simulink model "bidirectional_fixcurrent"  (R2016a)
settings: Solver=ode1  StartTime=0.0  StopTime=4  FixedStep=1e-5  RelTol=1e-3
undefined symbols (not defined in the file): Ion, Lithium
libraries: powerlib x12, simulink x4, powerlib_meascontrol x2, electricdrivelib x1
settings Model: Creator=CpmpuMark  LastModifiedBy=VARUN SINGH
settings DataIOCC: LimitDataPoints=on  SaveFormat=Array
settings DebuggingCC: SolverPrmCheckMsg=warning
settings HardwareCC: ProdBitPerPointer=32  ProdLargestAtomicFloat=None  ProdIntDivRoundTo=Undefined  ProdEndianess=Unspecified  ProdWordSize=32  ProdHWDeviceType=32-bit Generic
settings ModelReferenceCC: PropagateSignalLabelsOutOfModel=off
settings ConfigComp: CovSFcnEnable=off

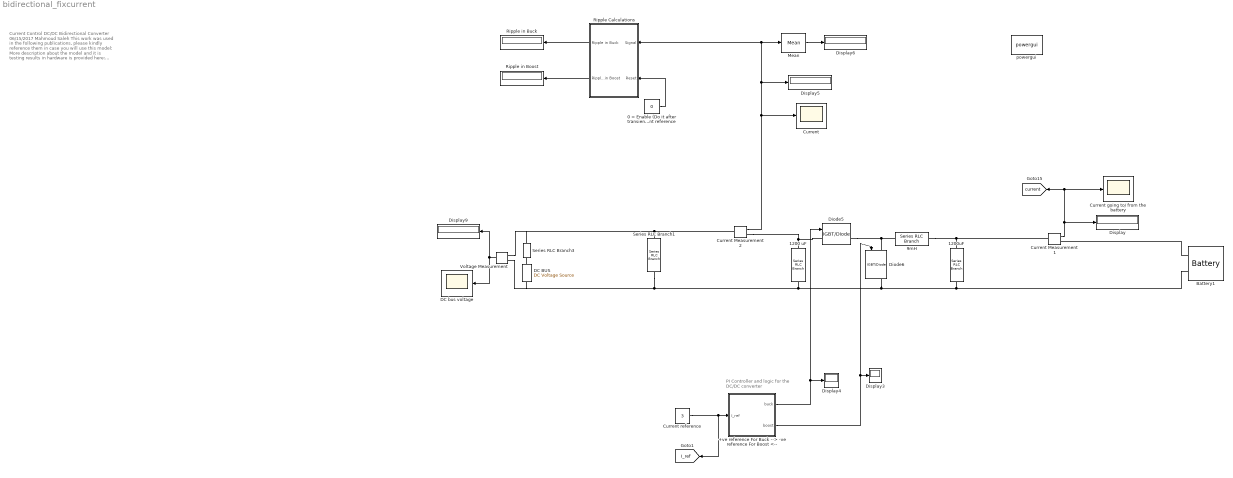
== system bidirectional_fixcurrent ==
  note: Current Control DC/DC Bidirectional Converter
      | 06/15/2017 Mahmoud Saleh
      | This work was used in the following publications, please kindly reference them in case you will use this model:
      |
      | More description about the model and it is testing results in hardware is provided here:
      | http://ieeexplore.ieee.org/document/7454295/
      | OR: https://drive.google.com/open?id=0B7mblFaJhY4VcmZ5OF9ueGxPM1U
      |
      | For Citation use :
      | - M. Saleh , Y. Esa, Y. Mhandi, W. Brandauer and A. Mohamed, "Design and implementation of CCNY DC microgrid testbed,"
      | 2016 IEEE Industry Applications Society Annual Meeting, Portland, OR, 2016.
      |
      | Also This Model was used in the paper:
      | http://ieeexplore.ieee.org/abstract/document/7731870/
      | OR: https://drive.google.com/open?id=0B7mblFaJhY4VY0dXdWdqTWNmUDg
      |
      | For Citation use :
      | -M. Saleh , A. Althaibani, Y. Esa, Y. Mhandi and A. Mohamed, "Impact of clustering microgrids on their stability and resilience during blackouts,"
      | 2015 International Conference on Smart Grid and Clean Energy Technologies (ICSGCE), Offenburg, 2015, pp. 195-200.
      |
      | The description of each element is on top of it and how it was calculated.
      | The model is flexible to work within wide range of values. If you have questions
      | please email me at my main email: mahmoudsah@hotmail.com
      | student email: msaleh000@citymail.cuny,edu
      | gmail: mahmoudsalahem@gmail.com
      | In the subject of your email write: Bidirectional Mathwork question
      | so that I would be able to track the emails even if they went to junk mail.
      | -------------------------------------------
      | I am an expert in modeling in Simulink, especially microgrids, I have encountered
      | many problems and I was able to fix it. I used to work with dSpace and I build with
      | my colleagues microgrid testbed at City College of New York. We modeled according
      | to the hardware components avialable in our lab, then we build it and test it. I
      | will try to help in case you have a question
  note: PI Controller and logic for
      | the DC/DC converter
  +ve reference For Buck --> -ve reference For Boost <-- : Subsystem
  "0 = Enable (Do it after transient, so that it does not calculate ripples during transient) 1 = Reset after every change in current reference" : Constant  Value=0
  1200 uF : powerlib/Elements/Series RLC Branch  LConnTagsString=__new0  RConnTagsString=__new0  BranchType=RC  Resistance=0.1  Inductance=3e-3  SetiL0=off  InitialCurrent=0  Capacitance=1200e-6  Setx0=off  InitialVoltage=0  Measurements=None
  1200uF : powerlib/Elements/Series RLC Branch  LConnTagsString=__new0  RConnTagsString=__new0  BranchType=C  Resistance=1  Inductance=3e-3  SetiL0=off  InitialCurrent=0  Capacitance=1200e-6  Setx0=off  InitialVoltage=0  Measurements=None
  9mH : powerlib/Elements/Series RLC Branch  LConnTagsString=__new0  RConnTagsString=__new0  BranchType=L  Resistance=1  Inductance=9e-3  SetiL0=off  InitialCurrent=0  Capacitance=1e-6  Setx0=off  InitialVoltage=0  Measurements=None
  Battery1 : electricdrivelib/Extra Sources/Battery  BatType=Lithium-Ion  ShowTempParam=off  ThermalPreset=no  NomV=120  NomQ=800  SOC=100  Batt_Tr=3  PresetModel=on  MaxQ=800  MinV=90  FullV=139.6785  Dis_rate=347.8261  R=0.0015  Normal_OP=723.4783  expZone="[129.6463      39.30435]"  current=[1.5 3]  Units=Ampere-hour  Tci=20  NomT=25  T2=0  MaxQ2=2.208  FullV2=3.45  Normal_OP2=2.8  expZone2="[3.22        0.23]"  Rca=0.6  ti=1000  Dp=0
  Current : Scope
  Current Measurement1 : powerlib/Measurements/Current Measurement  PhasorSimulation=off  OutputType=Complex  PSBequivalent=0
  Current Measurement2 : powerlib/Measurements/Current Measurement  PhasorSimulation=off  OutputType=Complex  PSBequivalent=0
  Current going to/ from the battery : Scope
  Current reference : Constant  Value=3
  DC BUS : powerlib/Electrical Sources/DC Voltage Source  Amplitude=300  Measurements=None
  DC bus voltage : Scope
  Diode5 : powerlib/Power Electronics/IGBT//Diode  Ron=1e-3  Rs=1e5  Cs=inf  Measurements=on
  Diode6 : powerlib/Power Electronics/IGBT//Diode  Ron=1e-3  Rs=1e5  Cs=inf  Measurements=on
  Display{,3..6,9} (6 alike) : Display
  Mean : powerlib_meascontrol/Measurements/Mean  Freq=10  Vinit=0  Ts=0
  Ripple Calculations : Subsystem
  Ripple in Boost : Display
  Ripple in Buck : Display
  Series RLC Branch1 : powerlib/Elements/Series RLC Branch  LConnTagsString=__new0  RConnTagsString=__new0  BranchType=R  Resistance=30  Inductance=3e-3  SetiL0=off  InitialCurrent=0  Capacitance=200e-6  Setx0=off  InitialVoltage=0  Measurements=None
  Series RLC Branch3 : powerlib/Elements/Series RLC Branch  LConnTagsString=__new0  RConnTagsString=__new0  BranchType=R  Resistance=1  Inductance=3e-3  SetiL0=off  InitialCurrent=0  Capacitance=200e-6  Setx0=off  InitialVoltage=0  Measurements=None
  Voltage Measurement : powerlib/Measurements/Voltage Measurement  PhasorSimulation=off  OutputType=Complex  PSBequivalent=0
  powergui : powerlib/powergui  Priority=1  SimulationMode=Discrete  SolverType=Backward Euler  SampleTime=1e-5  frequency=60  SPID=off  DisableSnubberDevices=off  DisableRonSwitches=off  DisableVfSwitches=off  SwTol=0  DisplayEquations=off  Interpol=off  ExternalGateDelay=off  methode=off  Ts=0  FunctionMessages=off  echomessages=off  HookPort=off  EnableUseOfTLC=off  x0status=blocks  frequencyindice=0  Pbase=100e6  ErrMax=1e-4  Iterations=50  UnitsV=kV  UnitsW=MW  buscounter=0  RestoreLinks=warning  ResistiveCurrentMeasurement=off  Frange=[0:2:500]  Ylog=off  Xlog=on  ShowGrid=off  save=off  variable=ZData  structure=0  ZoomFFT=off  StartTime=0.0  cycles=1  DisplayStyle=1  fundamental=60  FreqAxis=off  MaxFrequency=1000  frequencyindicesteady=1  RmsSteady=1  display=off
  tag scope: I_ref=global, current=global
  wires:
  Current Measurement1/1 -> [current], Current going to/ from the battery/1, Display/1
  +ve reference For Buck --> -ve reference For Boost <--/2(boost) -> Display3/1, Diode6/1
  Current reference/1 -> [I_ref], +ve reference For Buck --> -ve reference For Boost <--/1(I_ref)
  +ve reference For Buck --> -ve reference For Boost <--/1(buck) -> Display4/1, Diode5/1
  Voltage Measurement/1 -> Display9/1, DC bus voltage/1
  Current Measurement2/1 -> Current/1, Display5/1, Ripple Calculations/1(Signal), Mean/1
  Mean/1 -> Display6/1
  "0 = Enable (Do it after transient, so that it does not calculate ripples during transient) 1 = Reset after every change in current reference"/1 -> Ripple Calculations/2(Reset)
  Ripple Calculations/2(Ripple in Boost) -> Ripple in Boost/1
  Ripple Calculations/1(Ripple in Buck) -> Ripple in Buck/1
  connections:
  1200uF/RConn1 -- Battery1/LConn2 -- Diode6/RConn1 -- Voltage Measurement/LConn2 -- DC BUS/LConn1 -- Series RLC Branch1/RConn1 -- 1200 uF/RConn1
  Diode6/LConn1 -- Diode5/RConn1 -- 9mH/LConn1
  9mH/RConn1 -- Current Measurement1/LConn1 -- 1200uF/LConn1
  1200 uF/LConn1 -- Diode5/LConn1 -- Current Measurement2/RConn1
  Battery1/LConn1 -- Current Measurement1/RConn1
  Series RLC Branch1/LConn1 -- Current Measurement2/LConn1 -- Voltage Measurement/LConn1 -- Series RLC Branch3/LConn1
  Series RLC Branch3/RConn1 -- DC BUS/RConn1

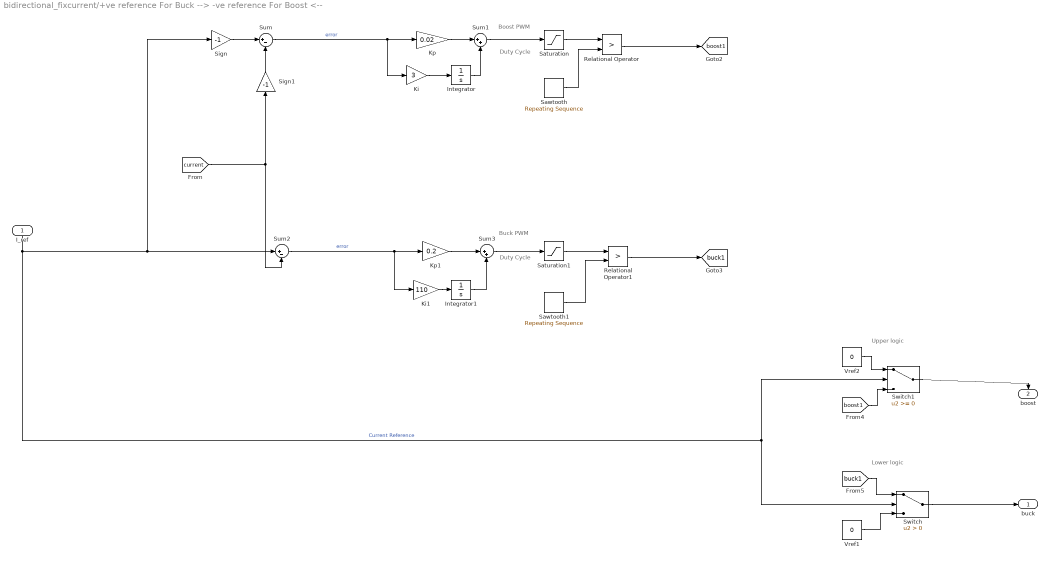
== system bidirectional_fixcurrent/+ve reference For Buck --> -ve reference For Boost <-- ==
  note: Buck PWM
  note: Duty Cycle
  note: Upper logic
  note: Lower logic
  note: Boost PWM
  note: Duty Cycle
  I_ref : Inport
  Integrator : Integrator  LimitOutput=on  UpperSaturationLimit=0.9  LowerSaturationLimit=0
  Integrator1 : Integrator  LimitOutput=on  UpperSaturationLimit=0.9  LowerSaturationLimit=0
  Ki : Gain  Gain=3
  Ki1 : Gain  Gain=110
  Kp : Gain  Gain=0.02
  Kp1 : Gain  Gain=0.2
  Relational Operator : RelationalOperator  Operator=>  OutDataTypeStr=boolean
  Relational Operator1 : RelationalOperator  Operator=>  OutDataTypeStr=boolean
  Saturation : Saturate  UpperLimit=0.9  LowerLimit=0
  Saturation1 : Saturate  UpperLimit=0.8  LowerLimit=0
  Sawtooth : simulink/Sources/Repeating Sequence  rep_seq_t=[0 1/5000]  rep_seq_y=[0 1]
  Sawtooth1 : simulink/Sources/Repeating Sequence  rep_seq_t=[0 1/5000]  rep_seq_y=[0 1]
  Sign : Gain  Gain=-1
  Sign1 : Gain  Gain=-1
  Sum : Sum  Inputs=|+-
  Sum1 : Sum  Inputs=|++
  Sum2 : Sum  Inputs=|+-
  Sum3 : Sum  Inputs=|++
  Switch : Switch  Criteria=u2 > Threshold
  Switch1 : Switch
  Vref1 : Constant  Value=0
  Vref2 : Constant  Value=0
  buck : Outport
  boost : Outport  Port=2
  tag scope: boost1=global, buck1=global
  wires:
  Integrator/1 -> Sum1/2
  Kp/1 -> Sum1/1
  Sum/1 -> Kp/1, Ki/1  "error"
  Relational Operator/1 -> [boost1]
  Sign/1 -> Sum/1
  Sum1/1 -> Saturation/1
  Ki/1 -> Integrator/1
  Sum3/1 -> Saturation1/1
  Integrator1/1 -> Sum3/2
  Sawtooth/1 -> Relational Operator/2
  Sawtooth1/1 -> Relational Operator1/2
  [current] -> Sum2/2, Sign1/1
  Kp1/1 -> Sum3/1
  Relational Operator1/1 -> [buck1]
  Sum2/1 -> Ki1/1, Kp1/1  "error"
  Saturation/1 -> Relational Operator/1
  Saturation1/1 -> Relational Operator1/1
  Ki1/1 -> Integrator1/1
  Switch1/1 -> boost/1
  Vref1/1 -> Switch/3
  Vref2/1 -> Switch1/1
  [boost1] -> Switch1/3
  Switch/1 -> buck/1
  [buck1] -> Switch/1
  I_ref/1 -> Sign/1, Sum2/1, Switch1/2, Switch/2  "Current Reference"
  Sign1/1 -> Sum/2

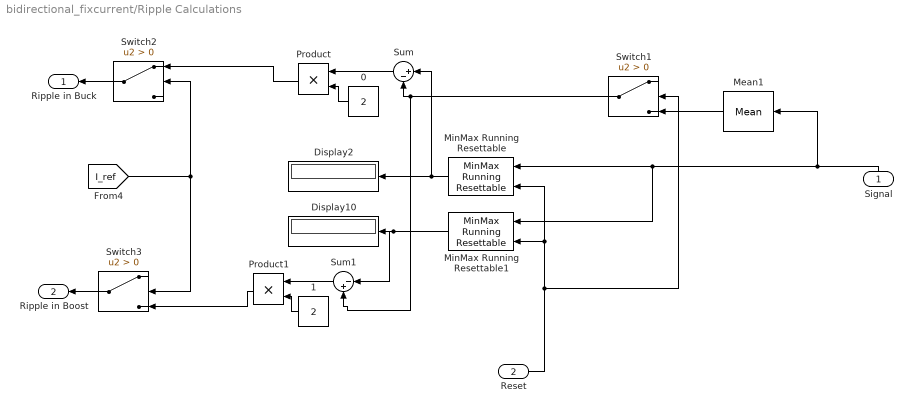
== system bidirectional_fixcurrent/Ripple Calculations ==
  Signal : Inport
  Reset : Inport  Port=2
  0 : Constant  Value=2
  1 : Constant  Value=2
  Display10 : Display
  Display2 : Display
  Mean1 : powerlib_meascontrol/Measurements/Mean  Freq=10  Vinit=0  Ts=0
  MinMax Running Resettable : simulink/Math Operations/MinMax Running Resettable  Function=max  vinit=0.0
  MinMax Running Resettable1 : simulink/Math Operations/MinMax Running Resettable  Function=min  vinit=0.0
  Product : Product
  Product1 : Product
  Sum : Sum  Inputs=|+-
  Sum1 : Sum  Inputs=|-+
  Switch1 : Switch  Criteria=u2 > Threshold
  Switch2 : Switch  Criteria=u2 > Threshold
  Switch3 : Switch  Criteria=u2 > Threshold
  Ripple in Buck : Outport
  Ripple in Boost : Outport  Port=2
  wires:
  1/1 -> Product1/2
  [I_ref] -> Switch2/2, Switch3/2
  Product1/1 -> Switch3/3
  0/1 -> Product/2
  Switch2/1 -> Ripple in Buck/1
  Switch3/1 -> Ripple in Boost/1
  Product/1 -> Switch2/1
  Signal/1 -> Mean1/1, MinMax Running Resettable1/1, MinMax Running Resettable/1
  Switch1/1 -> Sum1/2, Sum/2
  MinMax Running Resettable/1 -> Sum/1, Display2/1
  MinMax Running Resettable1/1 -> Sum1/1, Display10/1
  Sum/1 -> Product/1
  Reset/1 -> Switch1/2, MinMax Running Resettable1/2, MinMax Running Resettable/2
  Sum1/1 -> Product1/1
  Mean1/1 -> Switch1/3
